simulink model "straight_path"  (R2023b)
settings: Solver=FixedStepAuto  StartTime=0.0  StopTime=inf  FixedStep=0.002  RelTol=1e-3
model workspace (MAT data in the model file):
  SL_ROS_VariableLengthArrays_MaxSizes.CommonInfo.ArrayTruncateAction = 'EmitWarning'
  SL_ROS_VariableLengthArrays_MaxSizes.MsgTypeMap = containers.Map
  SL_ROS_VariableLengthArrays_MaxSizes.MsgTypeMap.serialization.keys = {'nav_msgs/Path'}
  SL_ROS_VariableLengthArrays_MaxSizes.MsgTypeMap.serialization.values{1}.PropertyName = 'poses'
  SL_ROS_VariableLengthArrays_MaxSizes.MsgTypeMap.serialization.values{1}.DataType = 'geometry_msgs/PoseStamped'
  SL_ROS_VariableLengthArrays_MaxSizes.MsgTypeMap.serialization.values{1}.MaxLength = 64
  SL_ROS_VariableLengthArrays_MaxSizes.MsgTypeMap.serialization.uniformity = 0
  SL_ROS_VariableLengthArrays_MaxSizes.MsgTypeMap.serialization.keyType = 'char'
  SL_ROS_VariableLengthArrays_MaxSizes.MsgTypeMap.serialization.valueType = 'any'
undefined symbols (not defined in the file): clock
libraries: ros2lib x8
settings Model: SimulationMode=external  Creator=ethan  LastModifiedBy=ethan
settings OptimizationCC: EnhancedBackFolding=on  PassReuseOutputArgsAs=Individual arguments  ZeroExternalMemoryAtStartup=off  ZeroInternalMemoryAtStartup=off  MaxStackSize=64  OptimizeBlockOrder=speed  DifferentSizesBufferReuse=on  OptimizationCustomize=off  EfficientTunableParamExpr=on
settings DebuggingCC: ParameterTunabilityLossMsg=error
settings HardwareCC: ProdBitPerLong=64  ProdHWDeviceType=Intel->x86-64 (Linux 64)
settings SFSimCC: MATLABDynamicMemAlloc=off
settings RTWCC: Description=Embedded Coder  SystemTargetFile=ert.tlc  HardwareBoard=Robot Operating System 2 (ROS 2)  TLCOptions="-aInlineSetEventsForThisBaseRateFcn=TLC_FALSE -aSuppressMultiTaskScheduler=TLC_FALSE  -aRateBasedStepFcn=0"  TemplateMakefile=ert_default_tmf  Toolchain=Colcon Tools  TargetLang=C++
settings CodeAppCC: ForceParamTrailComments=on  IgnoreCustomStorageClasses=off  OperatorAnnotations=on  SimulinkDataObjDesc=on  SFDataObjDesc=on  InsertBlockDesc=on
settings ERTTargetCC: CodeInterfacePackaging=C++ class  RootIOFormat=Structure reference

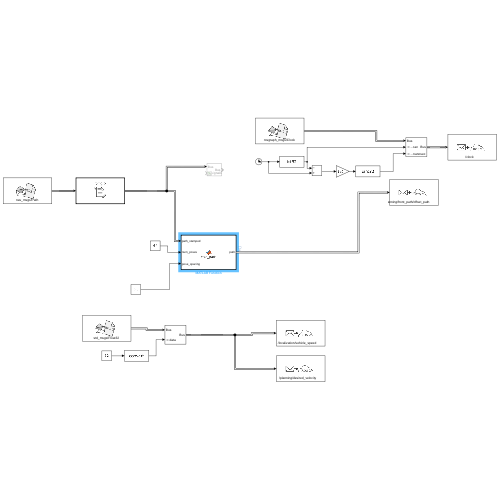
[thumbnail: Simulink's stored preview of the top-level diagram]
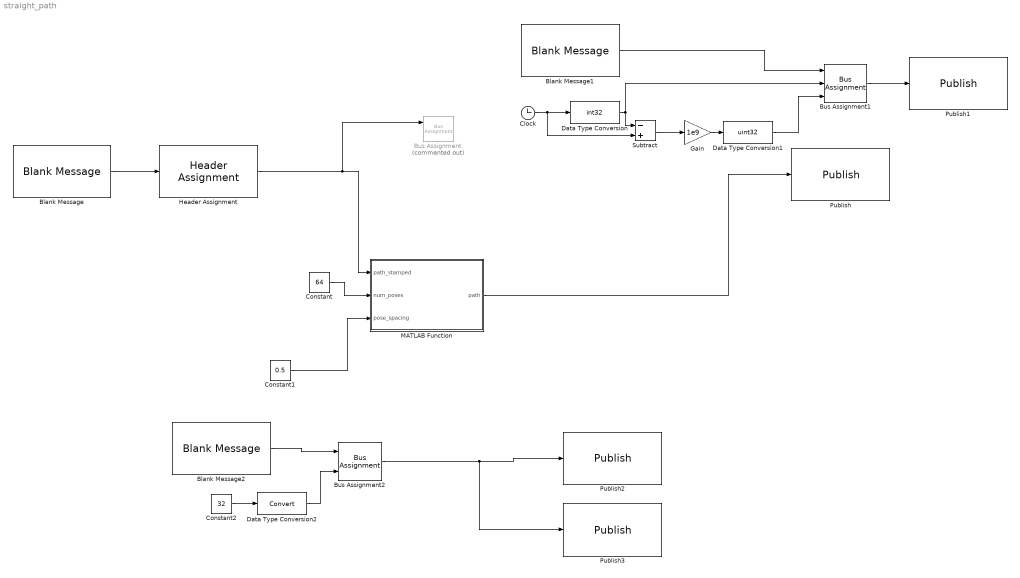
== system straight_path ==
  Blank Message : ros2lib/Blank Message  messageClass=Message  entityType=nav_msgs/Path  messageType=nav_msgs/Path  SampleTime=0.02
  Blank Message1 : ros2lib/Blank Message  messageClass=Message  entityType=rosgraph_msgs/Clock  messageType=rosgraph_msgs/Clock  SampleTime=-1
  Blank Message2 : ros2lib/Blank Message  messageClass=Message  entityType=std_msgs/Float32  messageType=std_msgs/Float32  SampleTime=0.01
  Bus Assignment : BusAssignment  Commented=on  AssignedSignals=signal1
  Bus Assignment1 : BusAssignment  AssignedSignals=clock.sec,clock.nanosec
  Bus Assignment2 : BusAssignment  AssignedSignals=data
  Clock : Clock
  Constant : Constant  Value=64
  Constant1 : Constant  Value=0.5
  Constant2 : Constant  Value=32
  Data Type Conversion : DataTypeConversion  OutDataTypeStr=int32  SaturateOnIntegerOverflow=off  RndMeth=Floor
  Data Type Conversion1 : DataTypeConversion  OutDataTypeStr=uint32  SaturateOnIntegerOverflow=off  RndMeth=Floor
  Data Type Conversion2 : DataTypeConversion  SaturateOnIntegerOverflow=off  RndMeth=Floor
  Gain : Gain  Gain=1e9
  Header Assignment : ros2lib/Header Assignment  SetFrameID=off  InsertTimeStamp=on  SetHeaderFieldName=Use the default header field name  HeaderFieldName=header
  MATLAB Function : MATLAB Function  TreatAsAtomicUnit=on
  Publish : ros2lib/Publish  topicSource=Select from ROS network  topic=/planning/front_path/offset_path  messageType=nav_msgs/Path  QOSHistory=Keep last  QOSDepth=1  QOSReliability=Reliable  QOSDurability=Volatile
  Publish1 : ros2lib/Publish  topicSource=Specify your own  topic=/clock  messageType=rosgraph_msgs/Clock  QOSHistory=Keep last  QOSDepth=1  QOSReliability=Reliable  QOSDurability=Volatile
  Publish2 : ros2lib/Publish  topicSource=Specify your own  topic=/localization/vehicle_speed  messageType=std_msgs/Float32  QOSHistory=Keep last  QOSDepth=1  QOSReliability=Reliable  QOSDurability=Volatile
  Publish3 : ros2lib/Publish  topicSource=Specify your own  topic=/planning/desired_velocity  messageType=std_msgs/Float32  QOSHistory=Keep last  QOSDepth=1  QOSReliability=Reliable  QOSDurability=Volatile
  Subtract : Sum  Inputs=-+
  wires:
  MATLAB Function/1(path) -> Publish/1
  Blank Message/1 -> Header Assignment/1
  Constant/1 -> MATLAB Function/2(num_poses)
  Constant1/1 -> MATLAB Function/3(pose_spacing)
  Header Assignment/1 -> Bus Assignment/1, MATLAB Function/1(path_stamped)
  Blank Message1/1 -> Bus Assignment1/1
  Clock/1 -> Data Type Conversion/1, Subtract/2
  Subtract/1 -> Gain/1
  Bus Assignment1/1 -> Publish1/1
  Data Type Conversion/1 -> Subtract/1, Bus Assignment1/2
  Gain/1 -> Data Type Conversion1/1
  Data Type Conversion1/1 -> Bus Assignment1/3
  Blank Message2/1 -> Bus Assignment2/1
  Constant2/1 -> Data Type Conversion2/1
  Bus Assignment2/1 -> Publish3/1, Publish2/1
  Data Type Conversion2/1 -> Bus Assignment2/2

== matlab function straight_path/MATLAB Function ==
  data: path_stamped input Bus: SL_Bus_nav_msgs_Path; path output Bus: SL_Bus_nav_msgs_Path; num_poses input; pose_spacing input
function path = calc_path(path_stamped, num_poses, pose_spacing)
path_stamped.poses_SL_Info.CurrentLength = uint32(num_poses);
%path_stamped.poses.header = path_stamped.header
x_coord = 0;
y_coord = 0;
for i = 1:num_poses
    path_stamped.poses(i).pose.position.x = x_coord;
    path_stamped.poses(i).pose.position.y = y_coord;
    path_stamped.poses(i).header = path_stamped.header
    x_coord = x_coord + pose_spacing;
    y_coord = y_coord + 0.5;
end

path = path_stamped;
